simulink model "FactorialUsingForLoop"  (R2021a)
settings: Solver=FixedStepDiscrete  StartTime=0.0  StopTime=10  RelTol=1e-3
settings Model: Creator=OmarMedhat  LastModifiedBy=OmarMedhat
settings OptimizationCC: DefaultParameterBehavior=Inlined  EnhancedBackFolding=on  PassReuseOutputArgsAs=Individual arguments  ZeroExternalMemoryAtStartup=off  ZeroInternalMemoryAtStartup=off  OptimizeBlockOrder=speed  DifferentSizesBufferReuse=on  OptimizationCustomize=off  EfficientTunableParamExpr=on
settings DebuggingCC: ParameterTunabilityLossMsg=error
settings SFSimCC: MATLABDynamicMemAlloc=off
settings RTWCC: SystemTargetFile=ert.tlc  GenCodeOnly=on  TemplateMakefile=ert_default_tmf  GenerateReport=on  IncludeHyperlinkInReport=on  LaunchReport=on  GenerateTraceInfo=on
settings CodeAppCC: ForceParamTrailComments=on  IgnoreCustomStorageClasses=off  OperatorAnnotations=on  SimulinkDataObjDesc=on  SFDataObjDesc=on  InsertBlockDesc=on
settings ERTTargetCC: TargetLangStandard=C99 (ISO)  GenerateSampleERTMain=on  InlinedParameterPlacement=NonHierarchical  ERTCustomFileTemplate=example_file_process.tlc

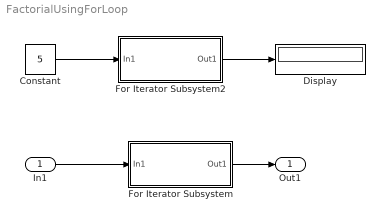
== system FactorialUsingForLoop ==
  In1 : Inport  OutDataTypeStr=uint16
  Constant : Constant  Value=5  OutDataTypeStr=uint16
  Display : Display
      settings: Format=decimal (Stored Integer)
  For Iterator Subsystem : Subsystem  TreatAsAtomicUnit=on
  For Iterator Subsystem2 : Subsystem  TreatAsAtomicUnit=on
  Out1 : Outport  OutDataTypeStr=uint16
  wires:
  For Iterator Subsystem/1(Out1) -> Out1/1
  In1/1 -> For Iterator Subsystem/1(In1)
  Constant/1 -> For Iterator Subsystem2/1(In1)
  For Iterator Subsystem2/1(Out1) -> Display/1

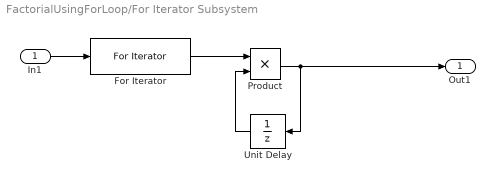
== system FactorialUsingForLoop/For Iterator Subsystem ==
  In1 : Inport
  For Iterator : ForIterator  IterationSource=external  IterationVariableDataType=uint16
  Product : Product  OutDataTypeStr=uint16
  Unit Delay : UnitDelay  InitialCondition=1  SampleTime=-1  HasFrameUpgradeWarning=on
  Out1 : Outport  OutDataTypeStr=uint16
  wires:
  For Iterator/1 -> Product/1
  Product/1 -> Unit Delay/1, Out1/1
  Unit Delay/1 -> Product/2
  In1/1 -> For Iterator/1

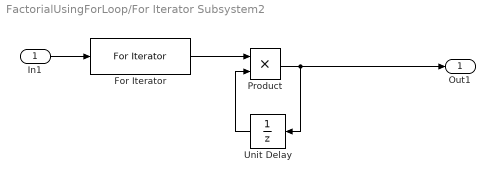
== system FactorialUsingForLoop/For Iterator Subsystem2 ==
  In1 : Inport
  For Iterator : ForIterator  IterationSource=external  IterationVariableDataType=uint16
  Product : Product  OutDataTypeStr=uint16
  Unit Delay : UnitDelay  InitialCondition=1  SampleTime=-1  HasFrameUpgradeWarning=on
  Out1 : Outport  OutDataTypeStr=uint16
  wires:
  For Iterator/1 -> Product/1
  Product/1 -> Unit Delay/1, Out1/1
  Unit Delay/1 -> Product/2
  In1/1 -> For Iterator/1
